simulink model "lab_6_task_1_simulink"  (R2025b)
settings: Solver=ode4  StartTime=0.0  StopTime=500  FixedStep=0.01  RelTol=1e-3
values from neighbouring files (symbols this model uses):
  ABN0 = eye(3)    [lab_6_task_1.m]    (also in lab_6_task_2.m)
  I = diag([ix iy iz])    [lab_4_task_1.m]    (also in lab_5_task_1.m; lab_5_task_2.m; lab_6_task_1.m = diag([ ix iy iz ]); lab_6_task_2.m = diag([ ix iy iz ]))
  n = sqrt(G*M_e/R^3)    [lab_6_task_1.m]    (also in lab_6_task_2.m; lab_7_task_1.m = sqrt(mu_E/(a^3)); lab_7_task_2.m = sqrt(mu_E/(a^3)); lab_7_task_3.m = sqrt(mu/(a^3)))
  w0 = [0.01 0.01 0.01]    [lab_3_task_3.m]    (also in lab_5_task_1.m = [wx0 wy0 wz0]; lab_5_task_2.m = [wx0 wy0 wz0]; lab_6_task_1.m = [wx0 wy0 wz0]; lab_6_task_2.m = [wx0 wy0 wz0])
  wLN = [0; 0; n;]    [lab_6_task_1.m]    (also in lab_6_task_2.m)
libraries: matrix_library x1
settings Model: Creator=nicol  LastModifiedBy=nicol

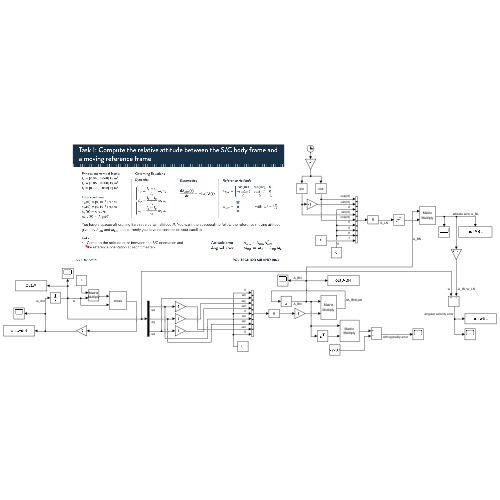
[thumbnail: Simulink's stored preview of the top-level diagram]
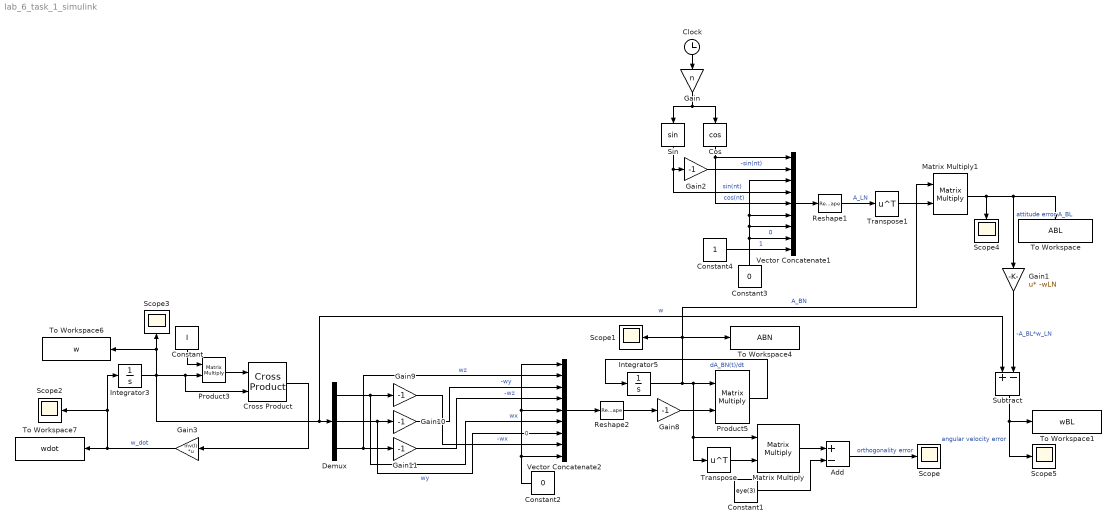
== system lab_6_task_1_simulink ==
  Add : Sum  Inputs=+-
  Clock : Clock
  Constant : Constant  Value=I
  Constant1 : Constant  Value=eye(3)
  Constant2 : Constant  Value=0
  Constant3 : Constant  Value=0
  Constant4 : Constant
  Cos : Trigonometry  Operator=cos
  Cross Product : matrix_library/Cross Product
  Demux : Demux  Outputs=3
  Gain : Gain  Gain=n
  Gain1 : Gain  Gain=-wLN  Multiplication=Matrix(u*K)
  Gain{2,8..11} (5 alike) : Gain  Gain=-1
  Gain3 : Gain  Gain=inv(I)  Multiplication=Matrix(K*u)
  Integrator3 : Integrator  InitialCondition=w0
  Integrator5 : Integrator  InitialCondition=ABN0
  Matrix Multiply : Product  Multiplication=Matrix(*)
  Matrix Multiply1 : Product  Multiplication=Matrix(*)
  Product3 : Product  Multiplication=Matrix(*)
  Product5 : Product  Multiplication=Matrix(*)
  Reshape1 : Reshape  OutputDimensionality=Customize  OutputDimensions=[3,3]
  Reshape2 : Reshape  OutputDimensionality=Customize  OutputDimensions=[3,3]
  Scope{,1..5} (6 alike) : Scope
      Scope settings: ActiveDisplayYMinimum=-6.807770444899007E-8  ActiveDisplayYMaximum=8.9871029145736092E-8
      Scope1 settings: ActiveDisplayYMinimum=-1.2493084857575658  ActiveDisplayYMaximum=1.2499231650841749
      Scope2 settings: ActiveDisplayYMinimum=-1  ActiveDisplayYMaximum=1  DataLoggingVariableName=ScopeData2
      Scope3 settings: ActiveDisplayYMinimum=-1  ActiveDisplayYMaximum=1  DataLoggingVariableName=ScopeData3
      Scope4 settings: ActiveDisplayYMinimum=-1  ActiveDisplayYMaximum=1  DataLoggingVariableName=ScopeData4
      Scope5 settings: ActiveDisplayYMinimum=-8.953871770327698  ActiveDisplayYMaximum=80.584845932949293  DataLoggingVariableName=ScopeData5
  Sin : Trigonometry
  Subtract : Sum  Inputs=+-
  To Workspace : ToWorkspace  VariableName=ABL  SaveFormat=Timeseries  SampleTime=-1
  To Workspace1 : ToWorkspace  VariableName=wBL  SaveFormat=Timeseries  SampleTime=-1
  To Workspace4 : ToWorkspace  VariableName=ABN  SaveFormat=Timeseries  SampleTime=-1
  To Workspace6 : ToWorkspace  VariableName=w  SaveFormat=Timeseries  SampleTime=-1
  To Workspace7 : ToWorkspace  VariableName=wdot  SaveFormat=Timeseries  SampleTime=-1
  Transpose : Math  Operator=transpose
  Transpose1 : Math  Operator=transpose
  Vector Concatenate1 : Concatenate  NumInputs=9
  Vector Concatenate2 : Concatenate  NumInputs=9
  wires:
  Gain9/1 -> Vector Concatenate2/8  "-wx"
  Cross Product/1 -> Gain3/1
  Gain8/1 -> Product5/2
  Product3/1 -> Cross Product/1
  Matrix Multiply/1 -> Add/1
  Integrator5/1 -> Matrix Multiply1/1, To Workspace4/1, Scope1/1, Transpose/1, Matrix Multiply/1, Product5/1  "A_BN"
  Demux/3 -> Vector Concatenate2/2, Gain11/1  "wz"
  Constant1/1 -> Add/2
  Vector Concatenate2/1 -> Reshape2/1
  Constant/1 -> Product3/1
  Reshape2/1 -> Gain8/1
  Gain11/1 -> Vector Concatenate2/4  "-wz"
  Add/1 -> Scope/1  "orthogonality error"
  Integrator3/1 -> Subtract/1, Demux/1, Cross Product/2, Product3/2, To Workspace6/1, Scope3/1  "w"
  Gain3/1 -> Scope2/1, Integrator3/1, To Workspace7/1  "w_dot"
  Demux/2 -> Vector Concatenate2/7, Gain10/1  "wy"
  Demux/1 -> Vector Concatenate2/6, Gain9/1  "wx"
  Product5/1 -> Integrator5/1  "dA_BN(t)/dt"
  Transpose/1 -> Matrix Multiply/2
  Constant2/1 -> Vector Concatenate2/1, Vector Concatenate2/5, Vector Concatenate2/9  "0"
  Gain10/1 -> Vector Concatenate2/3  "-wy"
  Vector Concatenate1/1 -> Reshape1/1
  Constant3/1 -> Vector Concatenate1/8, Vector Concatenate1/7, Vector Concatenate1/6, Vector Concatenate1/3  "0"
  Constant4/1 -> Vector Concatenate1/9  "1"
  Cos/1 -> Vector Concatenate1/5, Vector Concatenate1/1  "cos(nt)"
  Gain2/1 -> Vector Concatenate1/2  "-sin(nt)"
  Sin/1 -> Vector Concatenate1/4, Gain2/1  "sin(nt)"
  Reshape1/1 -> Transpose1/1  "A_LN"
  Transpose1/1 -> Matrix Multiply1/2
  Matrix Multiply1/1 -> Gain1/1, To Workspace/1, Scope4/1  "attitude error A_BL"
  Clock/1 -> Gain/1
  Gain/1 -> Sin/1, Cos/1
  Gain1/1 -> Subtract/2  "-A_BL*w_LN"
  Subtract/1 -> To Workspace1/1, Scope5/1  "angular velocity error"
